simulink model "experiment_supervisor_user"  (R2023b)
settings: Solver=FixedStepDiscrete  StartTime=0.0  StopTime=inf  FixedStep=1e-2  RelTol=1e-3
PreLoadFcn:
  | run('experiment_supervisor_data');
model workspace (MAT data in the model file):
  Ts = 0.01
undefined symbols (not defined in the file): current_target_timetable, ind, MCControlModes
libraries: dspswit3 x1, sldrtlib x1
settings Model: DataDictionary=EmbeddedBoardDD.sldd  Creator=mfussi  LastModifiedBy=mfussi
settings OptimizationCC: ReuseModelBlockBuffer=off  SimCompilerOptimization=on
settings DebuggingCC: ParameterPrecisionLossMsg=none  UnconnectedInputMsg=warning  UnconnectedOutputMsg=warning  UnconnectedLineMsg=warning
settings HardwareCC: ProdBitPerLong=64  ProdHWDeviceType=Intel->x86-64 (Linux 64)
settings ModelReferenceCC: EnableRefExpFcnMdlSchedulingChecks=on
settings RTWCC: Description=Simulink Desktop Real-Time  SystemTargetFile=sldrt.tlc  TemplateMakefile=sldrt.tmf  TargetLang=C++  RTWCompilerOptimization=on  DLArmComputeVersion=19.05
settings CodeAppCC: MaxIdLength=95
settings SimulinkDesktopRealTimeCC: TargetLibSuffix=_sldrt.a  TargetPreCompLibLocation=C:\Program Files\MATLAB\R2023b\toolbox\sldrt\lib\win64  TargetLangStandard=C++11 (ISO)

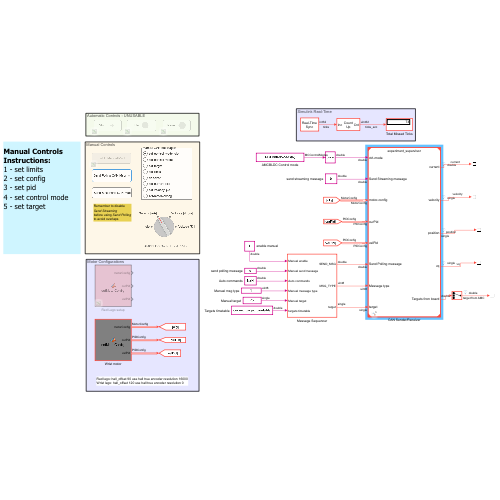
[thumbnail: Simulink's stored preview of the top-level diagram]
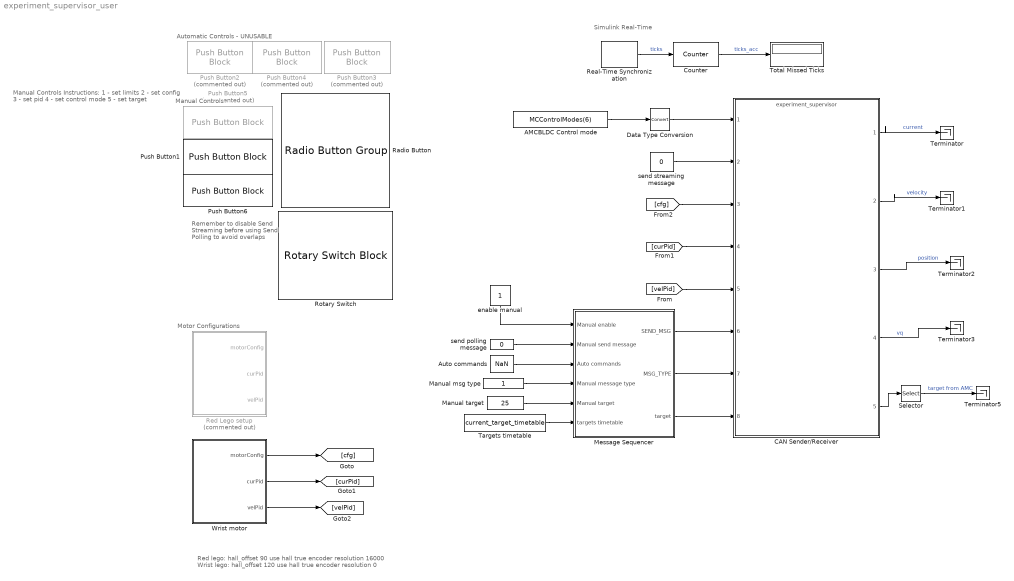
== system experiment_supervisor_user ==
  note: Manual Controls Instructions:
      | 1 - set limits
      | 2 - set config
      | 3 - set pid
      | 4 - set control mode
      | 5 - set target
  note: Motor Configurations
  note: Red lego: hall_offset 90 use hall true encoder resolution 16000
      | Wrist lego: hall_offset 120 use hall true encoder resolution 0
  note: Remember to disable
      | Send Streaming
      | before using Send Polling
      | to avoid overlaps
  note: Simulink Real-Time
  note: Manual Controls
  note: Automatic Controls - UNUSABLE
  AMCBLDC Control mode : Constant  Value=MCControlModes(6)
  Auto commands : Constant  Value=NaN
  CAN Sender/Receiver : ModelReference  ModelNameDialog=experiment_supervisor.slx  SimulationMode=Normal  ModelReferenceVersion=5.17
  Counter : dspswit3/Counter  Direction=Up  CountEvent=Rising edge  CounterSize=32 bits  MaxCount=255  InitialCount=0  Output=Count  HitValue=32  ResetInput=off  SamplesPerFrame=1  Ts=1  CntDtype=uint32  HitDtype=Logical
  Data Type Conversion : DataTypeConversion  SaturateOnIntegerOverflow=off  RndMeth=Floor
  Manual msg type : Constant  OutDataTypeStr=uint8
  Manual target : Constant  Value=25  OutDataTypeStr=single
  Message Sequencer : Subsystem
  Push Button1 : PushButtonBlock  ButtonText=Send Polling CAN Msg  Icon=Triangle  IconAlignment=Right  IconColor=On  OffValue=0.000000
  Push Button2 : PushButtonBlock  Commented=on  ButtonText=Start  Icon=TurnSignalRight  IconAlignment=Right  IconColor=On  OffValue=-nan(ind)
  Push Button3 : PushButtonBlock  Commented=on  ButtonText=Reset  OnValue=2  Icon=Hexagon  IconAlignment=Right  IconColor=On  OffValue=2.000000
  Push Button4 : PushButtonBlock  Commented=on  ButtonText=Idle  OnValue=0  Icon=Circle  IconAlignment=Right  IconColor=On  OffValue=-1.000000
  Push Button5 : PushButtonBlock  Commented=on  ButtonText=Enable Manual Mode  ButtonType=Latch  IconAlignment=Right  OffValue=0.000000
  Push Button6 : PushButtonBlock  ButtonText=Send Streaming CAN Msg  ButtonType=Latch  Icon=TurnSignalRight  IconAlignment=Right  IconColor=On  OffValue=0.000000
  Radio Button : RadioButtonGroup  LabelPosition=Hide  SelectedLabel=set-control-mode-idle  ButtonGroupName=Manual CAN Messages
      settings: Values={{'set-control-mode-idle', 'set-control-mode', 'set-target', 'set-limits', 'discover', 'set-current-pid', 'set-velocity-pid', 'set-motor-config'}, [1 2 3 4 5 6 7 8]}
  Real-Time Synchronization : sldrtlib/Real-Time Synchronization  SampleTime=Ts  MaxMissedTicks=inf  ShowMissedTicks=on  YieldWhenWaiting=off
  Red Lego setup : MATLAB Function  Commented=on  TreatAsAtomicUnit=on
  Rotary Switch : RotarySwitchBlock  LabelPosition=Bottom
      settings: Values={{'Idle', 'Current [mA]', 'Velocity [deg/s]', 'Voltage [%]'}, [0 6 10 80]}
  Selector : Selector  InputPortWidth=3  IndexOptions=Index vector (dialog)  Indices=[1]  OutputSizes=1
  Targets timetable : Constant  Value=current_target_timetable
  Terminator{,1..3,5} (5 alike) : Terminator
  Total Missed Ticks : Display
      settings: Decimation=5
  Wrist motor : MATLAB Function  TreatAsAtomicUnit=on
  enable manual : Constant
  send polling message : Constant  Value=0
  send streaming message : Constant  Value=0
  wires:
  Real-Time Synchronization/1 -> Counter/1  "ticks"
  Counter/1 -> Total Missed Ticks/1  "ticks_acc"
  CAN Sender/Receiver/1 -> Terminator/1  "current"
  CAN Sender/Receiver/4 -> Terminator3/1  "vq"
  CAN Sender/Receiver/2 -> Terminator1/1  "velocity"
  CAN Sender/Receiver/3 -> Terminator2/1  "position"
  AMCBLDC Control mode/1 -> Data Type Conversion/1
  Data Type Conversion/1 -> CAN Sender/Receiver/1
  CAN Sender/Receiver/5 -> Selector/1
  Selector/1 -> Terminator5/1  "target from AMC"
  Wrist motor/1(motorConfig) -> [cfg]
  Wrist motor/2(curPid) -> [curPid]
  Wrist motor/3(velPid) -> [velPid]
  [velPid] -> CAN Sender/Receiver/5
  [curPid] -> CAN Sender/Receiver/4
  [cfg] -> CAN Sender/Receiver/3
  send streaming message/1 -> CAN Sender/Receiver/2
  Message Sequencer/3(target) -> CAN Sender/Receiver/8
  Message Sequencer/1(SEND_MSG) -> CAN Sender/Receiver/6
  Message Sequencer/2(MSG_TYPE) -> CAN Sender/Receiver/7
  enable manual/1 -> Message Sequencer/1(Manual enable)
  Manual target/1 -> Message Sequencer/5(Manual target)
  send polling message/1 -> Message Sequencer/2(Manual send message)
  Manual msg type/1 -> Message Sequencer/4(Manual message type)
  Auto commands/1 -> Message Sequencer/3(Auto commands)
  Targets timetable/1 -> Message Sequencer/6(targets timetable)

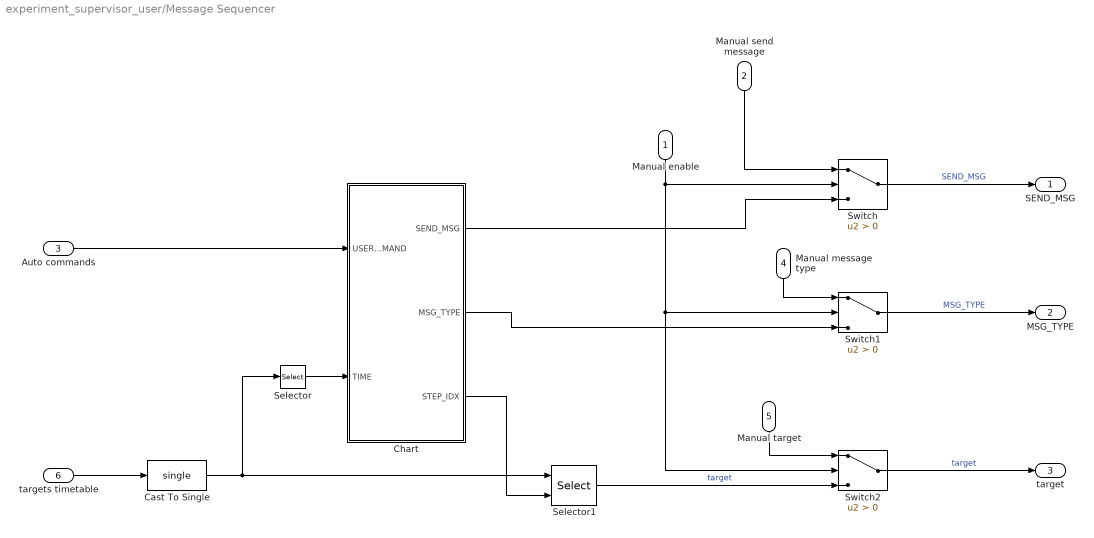
== system experiment_supervisor_user/Message Sequencer ==
  Manual enable : Inport
  Manual send message : Inport  Port=2
  Auto commands : Inport  Port=3
  Manual message type : Inport  Port=4
  Manual target : Inport  Port=5
  targets timetable : Inport  Port=6
  Cast To Single : DataTypeConversion  OutDataTypeStr=single  SaturateOnIntegerOverflow=off  RndMeth=Floor
  Chart : Stateflow chart  TreatAsAtomicUnit=on
      settings: PortSchema="{\"entries\":[{\"content\":{\"sides\":[{\"content\":{\"connectorIds\":[\"In1\",\"In2\"]},\"type\":\"ConnectorPlacement.EquallySpacedRectSide\",\"uuid\":\"3f3ecf7a-eca8-49e2-a594-4c8df01bcae2\"},{\"content\":{\"connectorIds\":[\"Out2\",\"Out1\",\"Out3\"],\"side\":\"RIGHT\"},\"type\":\"ConnectorPlacement.EquallySpacedRectSide\",\"uuid\":\"2e405059-6050-4daf-b42b-e1c8d6f3a572\"},{\"content\":{\"connectorIds\":[],\"side\":\"TOP\"},\"type\":\"ConnectorPlacement.EquallySpacedRectSide\",\"uuid\":\"8705f6e5-e301-4990-b24d-44270950b42f\"}]},\"type\":\"ConnectorPlacement.EquallySpacedConnector\",\"uuid\":\"46b9b7aa-14e0-48f8-b8fe-455c7835f2bb\"}],\"packageUris\":[\"http://schema.mathworks.com/mf0/Connector/R2020b\"],\"version\":\"1.0\"}"
  Selector : Selector  NumberOfDimensions=2  InputPortWidth=2  IndexOptions=Index vector (dialog),Select all  Indices=1,2  OutputSizes=1,6
  Selector1 : Selector  NumberOfDimensions=2  InputPortWidth=2  IndexOptions=Index vector (dialog),Index vector (port)  Indices=2,2  OutputSizes=1,6
  Switch : Switch  Criteria=u2 > Threshold  SaturateOnIntegerOverflow=off  InputSameDT=off
  Switch1 : Switch  Criteria=u2 > Threshold  SaturateOnIntegerOverflow=off  InputSameDT=off
  Switch2 : Switch  Criteria=u2 > Threshold  SaturateOnIntegerOverflow=off  InputSameDT=off
  SEND_MSG : Outport
  MSG_TYPE : Outport  Port=2
  target : Outport  Port=3
  wires:
  Manual enable/1 -> Switch1/2, Switch2/2, Switch/2
  Selector/1 -> Chart/2(TIME)
  Chart/3(STEP_IDX) -> Selector1/2
  Selector1/1 -> Switch2/3  "target"
  Manual target/1 -> Switch2/1
  Chart/1(MSG_TYPE) -> Switch1/3
  Switch2/1 -> target/1  "target"
  Chart/2(SEND_MSG) -> Switch/3
  targets timetable/1 -> Cast To Single/1
  Manual send message/1 -> Switch/1
  Switch/1 -> SEND_MSG/1  "SEND_MSG"
  Auto commands/1 -> Chart/1(USER_COMMAND)
  Manual message type/1 -> Switch1/1
  Switch1/1 -> MSG_TYPE/1  "MSG_TYPE"
  Cast To Single/1 -> Selector/1, Selector1/1

== matlab function experiment_supervisor_user/Wrist motor ==
  data: motorConfig output Bus: MotorConfig; curPid output Bus: PIDConfig; velPid output Bus: PIDConfig
function [motorConfig, curPid, velPid] = setMotorConfig()

motorConfig.hall_sens_offset = single(30); % deg
motorConfig.has_hall_sens = true;
motorConfig.has_quadrature_encoder = false;
motorConfig.has_speed_quadrature_encoder = false;
motorConfig.has_torque_sens = false;
motorConfig.use_index = false;
motorConfig.enable_verbosity = true;
motorConfig.rotor_encoder_resolution = int16(0); % set to 0 to use only hall sensors
motorConfig.rotor_index_offset = int16(0);
motorConfig.encoder_tolerance = uint8(0);
motorConfig.pole_pairs = uint8(7);
motorConfig.Kbemf = single(0);
motorConfig.Rphase = single(0);
motorConfig.Imin = single(-1e3);
motorConfig.Imax = single(1e3);
motorConfig.Vmax = single(24);
motorConfig.resistance = single(25.9);
motorConfig.inductance = single(271);
motorConfig.thermal_resistance = single(56);
motorConfig.thermal_time_constant = single(270);

% Hall offset and BC phases swap is not available as a CAN message
% The parameters need to be changed in rtw_motor_config.c
swap_bc = 1;

% ---------------------------------

curPid.OutMax = single(100);
curPid.OutMin = single(-100);
curPid.P = single(2);
curPid.I = single(500);
curPid.D = single(0);
curPid.N = single(100);
curPid.I0 = single(0);
curPid.D0 = single(0);
curPid.shift_factor = uint8(0);


velPid.OutMax = single(1000);
velPid.OutMin = single(-1000);
velPid.P = single(-1000);
velPid.I = single(-1000);
velPid.D = single(0);
velPid.N = single(100);
velPid.I0 = single(0);
velPid.D0 = single(0);
velPid.shift_factor = uint8(10);

== matlab function experiment_supervisor_user/Red Lego setup ==
  data: motorConfig output Bus: MotorConfig; curPid output Bus: PIDConfig; velPid output Bus: PIDConfig
function [motorConfig, curPid, velPid] = setMotorConfig()

motorConfig.hall_sens_offset = single(30); % deg
motorConfig.has_hall_sens = true;
motorConfig.has_quadrature_encoder = true;
motorConfig.has_speed_quadrature_encoder = false;
motorConfig.has_torque_sens = false;
motorConfig.use_index = false;
motorConfig.enable_verbosity = true;
motorConfig.rotor_encoder_resolution = int16(16000);
motorConfig.rotor_index_offset = int16(0);
motorConfig.encoder_tolerance = uint8(0);
motorConfig.pole_pairs = uint8(4);
motorConfig.Kbemf = single(0);
motorConfig.Rphase = single(0);
motorConfig.Imin = single(-1e3);
motorConfig.Imax = single(1e3);
motorConfig.Vcc = single(24);
motorConfig.Vmax = single(24);

% Hall offset and BC phases swap is not available as a CAN message
% The parameters need to be changed in rtw_motor_config.c
swap_bc = 1;

% ---------------------------------

curPid.OutMax = single(100);
curPid.OutMin = single(-100);
curPid.P = single(2);
curPid.I = single(500);
curPid.D = single(0);
curPid.N = single(100);
curPid.I0 = single(0);
curPid.D0 = single(0);
curPid.shift_factor = uint8(0);


velPid.OutMax = single(1000);
velPid.OutMin = single(-1000);
velPid.P = single(1000);
velPid.I = single(1000);
velPid.D = single(0);
velPid.N = single(100);
velPid.I0 = single(0);
velPid.D0 = single(0);
velPid.shift_factor = uint8(10);

== stateflow chart experiment_supervisor_user/Message Sequencer/Chart ==
  state RESET_IDLE
    entry:
    SEND_MSG=1;
    STEP_IDX=1;
    on after(1, sec):
    SEND_MSG=0;
  state WAIT_LIMITS
    entry:
    SEND_MSG=1;
    on after(1, sec):
    SEND_MSG=0;
  state IDLE
    entry:
    SEND_MSG=1;
    STEP_IDX=1;
    on after(1 , sec):
    SEND_MSG=0;
  state STARTED
    entry:
    SEND_MSG=1;
    on after(1 , sec):
    SEND_MSG=0;
  state WAIT_CTRL_MODE
    entry:
    SEND_MSG=1;
    on after(1,sec):
    SEND_MSG=0;
  (default) -> RESET_IDLE
  STARTED -> RESET_IDLE [order 4] : [USER_COMMAND == 2]
      | {MSG_TYPE = 1;}
  RESET_IDLE -> WAIT_LIMITS [order 1] : [USER_COMMAND == 1]
      | {MSG_TYPE = 4;}
  IDLE -> RESET_IDLE [order 2] : [USER_COMMAND == 2]
      | {MSG_TYPE=1;}
  WAIT_LIMITS -> RESET_IDLE [order 2] : [USER_COMMAND == 2]
      | {MSG_TYPE = 1;}
  RESET_IDLE -> RESET_IDLE [order 2] : [USER_COMMAND == 2]
      | {MSG_TYPE=1;}
  WAIT_CTRL_MODE -> RESET_IDLE [order 2] : [USER_COMMAND == 2]
      | {MSG_TYPE = 1;}
  IDLE -> IDLE [order 3] : [USER_COMMAND == 0 ]
      | {MSG_TYPE=1;}
  WAIT_LIMITS -> WAIT_CTRL_MODE [order 1] : after(2, sec){MSG_TYPE = 2;}
  STARTED -> IDLE [order 2] : [USER_COMMAND == 0 ]
      | {MSG_TYPE=1;}
  IDLE -> WAIT_CTRL_MODE [order 1] : [USER_COMMAND == 1]
      | {MSG_TYPE = 2;}
  WAIT_CTRL_MODE -> STARTED [order 1] : after(2, sec){MSG_TYPE=3;
      | STEP_IDX=1;}
  STARTED -> STARTED [order 1] : after(TIME(STEP_IDX), sec)[STEP_IDX <length(TIME)]
      | {STEP_IDX = STEP_IDX + 1;}
  STARTED -> STARTED [order 3] : [USER_COMMAND == 1]{MSG_TYPE = 3;}
  data: MSG_TYPE output uint8 =uint8(1); USER_COMMAND input; SEND_MSG output uint8 =uint8(0); TIME input; STEP_IDX output uint32 =uint32(1)
